simulink model "Week2"  (R2023b)
settings: Solver=ode1  StartTime=0.0  StopTime=25  FixedStep=dT_current  RelTol=1e-3
values from neighbouring files (symbols this model uses):
  A_current = current_values.(4)    [Week2_Code_V2.m]    (also in Week2_code.m)
  b_current = current_values.(3)    [Week2_Code_V2.m]    (also in Week2_code.m)
  freq_current = current_values.(5)    [Week2_Code_V2.m]    (also in Week2_code.m)
  J_current = current_values.(2)    [Week2_Code_V2.m]    (also in Week2_code.m)
  w_0_current = current_values.(1)    [Week2_Code_V2.m]    (also in Week2_code.m)
settings Model: Creator=jessi  LastModifiedBy=jessi

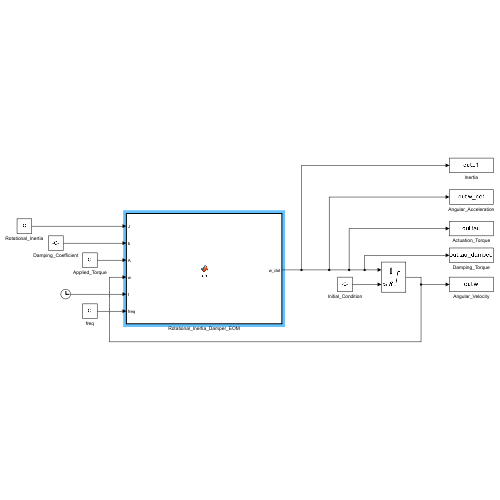
[thumbnail: Simulink's stored preview of the top-level diagram]
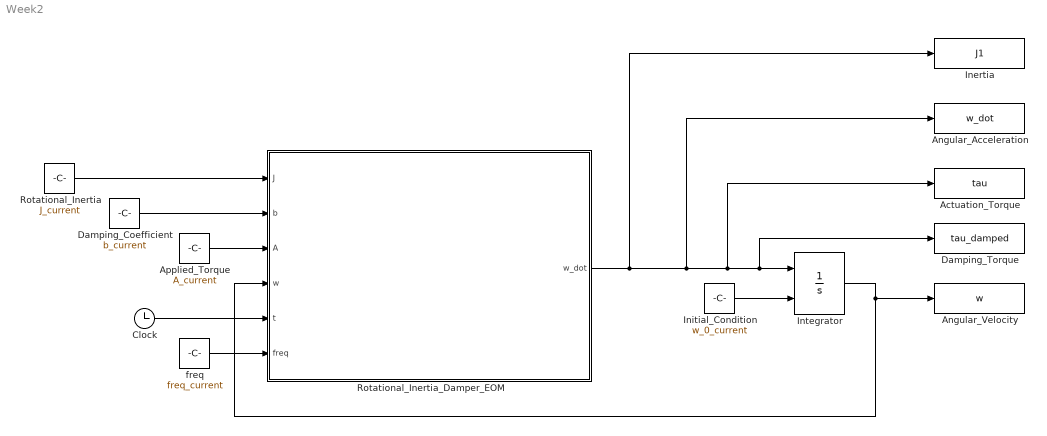
== system Week2 ==
  Actuation_Torque : ToWorkspace  VariableName=tau  SaveFormat=Timeseries  SampleTime=-1
  Angular_Acceleration : ToWorkspace  VariableName=w_dot  SaveFormat=Timeseries  SampleTime=-1
  Angular_Velocity : ToWorkspace  VariableName=w  SaveFormat=Timeseries  SampleTime=-1
  Applied_Torque : Constant  Value=A_current
  Clock : Clock
  Damping_Coefficient : Constant  Value=b_current
  Damping_Torque : ToWorkspace  VariableName=tau_damped  SaveFormat=Timeseries  SampleTime=-1
  Inertia : ToWorkspace  VariableName=J1  SaveFormat=Timeseries  SampleTime=-1
  Initial_Condition : Constant  Value=w_0_current
  Integrator : Integrator  InitialConditionSource=external  LimitOutput=on  UpperSaturationLimit=100
  Rotational_Inertia : Constant  Value=J_current
  Rotational_Inertia_Damper_EOM : MATLAB Function  TreatAsAtomicUnit=on
  freq : Constant  Value=freq_current
  wires:
  Rotational_Inertia/1 -> Rotational_Inertia_Damper_EOM/1(J)
  Damping_Coefficient/1 -> Rotational_Inertia_Damper_EOM/2(b)
  Applied_Torque/1 -> Rotational_Inertia_Damper_EOM/3(A)
  Rotational_Inertia_Damper_EOM/1(w_dot) -> Inertia/1, Integrator/1, Damping_Torque/1, Actuation_Torque/1, Angular_Acceleration/1
  Initial_Condition/1 -> Integrator/2
  Clock/1 -> Rotational_Inertia_Damper_EOM/5(t)
  Integrator/1 -> Angular_Velocity/1, Rotational_Inertia_Damper_EOM/4(w)
  freq/1 -> Rotational_Inertia_Damper_EOM/6(freq)

== matlab function Week2/Rotational_Inertia_Damper_EOM ==
  data: J input; w_dot output; b input; A input; w input; t input; freq input
function w_dot = fcn(J,b,A,w,t,freq)

tau_damped = b*w;
tau = A*sin(w*t);
w_dot = (1/J)*(A-b*w);
J1 = (tau-tau_damped)/(w_dot);

end
